simulink model "quadrotor_r2022b"  (R2022b)
settings: Solver=ode4  StartTime=0.0  StopTime=60  FixedStep=1e-3  RelTol=1e-3
libraries: slpidlib x10, dspindex x6, sharedtransform x3, simulink x3, shared6dof x1
(part 2 of 2)

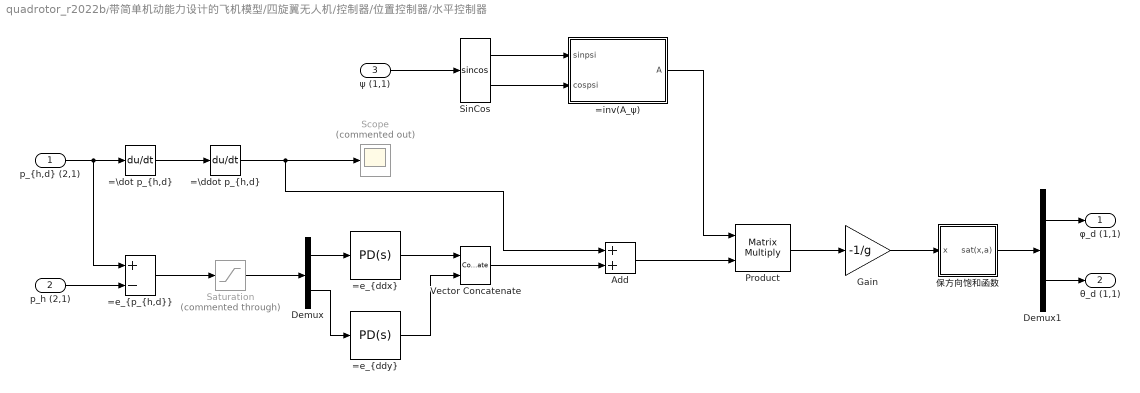
== system quadrotor_r2022b/带简单机动能力设计的飞机模型/四旋翼无人机/控制器/位置控制器/水平控制器 ==
  "p_{h,d} (2,1)" : Inport
  p_h (2,1) : Inport  Port=2
  ψ (1,1) : Inport  Port=3
  "=\\ddot p_{h,d}" : Derivative
  "=\\dot p_{h,d}" : Derivative
  "=e_{ddx}" : slpidlib/PID Controller  Controller=PD  Form=Parallel  TimeDomain=Continuous-time  UseExternalTs=off  SampleTime=-1  IntegratorMethod=Forward Euler  FilterMethod=Forward Euler  ControllerParametersSource=internal  P=K_P_h  I=0  UseKiTs=off  D=K_D_h  N=K_N_h  UseFilter=on  TunerSelectOption=Transfer Function Based (PID Tuner App)  InitialConditionSource=internal  InitialConditionForIntegrator=0  InitialConditionForFilter=0  DifferentiatorICPrevScaledInput=0  ExternalReset=none  TrackingMode=off  Kt=1  LimitOutput=off  SatLimitsSource=internal  UpperSaturationLimit=inf  LowerSaturationLimit=-inf  LinearizeAsGain=on  AntiWindupMode=none  Kb=1  LimitIntegrator=off  UpperIntegratorSaturationLimit=inf  LowerIntegratorSaturationLimit=-inf  POutMin=[]  POutMax=[]  IOutMin=[]  IOutMax=[]  DOutMin=[]  DOutMax=[]  NOutMin=[]  NOutMax=[]  SumOutMin=[]  SumOutMax=[]  SaturationOutMin=[]  SaturationOutMax=[]  PParamMin=[]  PParamMax=[]  IParamMin=[]  IParamMax=[]  DParamMin=[]  DParamMax=[]  NParamMin=[]  NParamMax=[]  KbParamMin=[]  KbParamMax=[]  KtParamMin=[]  KtParamMax=[]  KbOutMin=[]  KbOutMax=[]  KtOutMin=[]  KtOutMax=[]  IntegratorOutMin=[]  IntegratorOutMax=[]  FilterOutMin=[]  FilterOutMax=[]  SumI1OutMin=[]  SumI1OutMax=[]  SumI2OutMin=[]  SumI2OutMax=[]  SumI3OutMin=[]  SumI3OutMax=[]  SumI4OutMin=[]  SumI4OutMax=[]  SumDOutMin=[]  SumDOutMax=[]  DifferentiatorOutMin=[]  DifferentiatorOutMax=[]  FilterDiffOutCoefMin=[]  FilterDiffOutCoefMax=[]  ReciprocalOutMin=[]  ReciprocalOutMax=[]  SumDenOutMin=[]  SumDenOutMax=[]  SumNumOutMin=[]  SumNumOutMax=[]  DivideOutMin=[]  DivideOutMax=[]  UdiffTsProdOutMin=[]  UdiffTsProdOutMax=[]  NTsProdOutMin=[]  NTsProdOutMax=[]  UintegralTsProdOutMin=[]  UintegralTsProdOutMax=[]  UngainTsProdOutMin=[]  UngainTsProdOutMax=[]  ClampingZeroOutDataTypeStr=Inherit: Inherit via back propagation  ClampingZeroOutMin=[]  ClampingZeroOutMax=[]  FilterDenConstantOutDataTypeStr=Inherit: Inherit via back propagation  FilterDenConstantOutMin=[]  FilterDenConstantOutMax=[]  PCopyOutDataTypeStr=Inherit: Inherit via back propagation  PCopyOutMin=[]  PCopyOutMax=[]  NCopyOutDataTypeStr=Inherit: Inherit via back propagation  NCopyOutMin=[]  NCopyOutMax=[]  IntegratorContinuousStateAttributes=''  IntegratorStateMustResolveToSignalObject=off  IntegratorRTWStateStorageClass=Auto  FilterContinuousStateAttributes=''  FilterStateMustResolveToSignalObject=off  FilterRTWStateStorageClass=Auto  ParallelPVariant=InternalParameters  IdealPVariant=Disabled  IVariant=Disabled  DVariant=InternalParameters  IntegratorVariant=Disabled  SatVariant=Disabled  AWVariant=Disabled  PCopyVariant=Disabled  TRVariant=Disabled  FdbkBlocksVariant=Forward  IdealPFdbkVariant=Disabled  SatFdbkVariant=Disabled  DerivativeFilterVariant=ContFilter  NVariant=InternalParameters  NCopyVariant=Disabled  FilterICVariant=InternalICsFilter  IntegratorICVariant=Disabled  ExternalResetVariant=Disabled  TRSumVariant=Passthrough  SumFdbkVariant=Disabled  SumVariant=Sum_PD  TsampFilterVariant=InternalTs  TsampNgainVariant=Passthrough  TsampIntegralVariant=Disabled_SignalSpec  ExternalSaturationOutDataTypeStr=Inherit: Same as second input
  "=e_{ddy}" : slpidlib/PID Controller  Controller=PD  Form=Parallel  TimeDomain=Continuous-time  UseExternalTs=off  SampleTime=-1  IntegratorMethod=Forward Euler  FilterMethod=Forward Euler  ControllerParametersSource=internal  P=K_P_h  I=0  UseKiTs=off  D=K_D_h  N=K_N_h  UseFilter=on  TunerSelectOption=Transfer Function Based (PID Tuner App)  InitialConditionSource=internal  InitialConditionForIntegrator=0  InitialConditionForFilter=0  DifferentiatorICPrevScaledInput=0  ExternalReset=none  TrackingMode=off  Kt=1  LimitOutput=off  SatLimitsSource=internal  UpperSaturationLimit=inf  LowerSaturationLimit=-inf  LinearizeAsGain=on  AntiWindupMode=none  Kb=1  LimitIntegrator=off  UpperIntegratorSaturationLimit=inf  LowerIntegratorSaturationLimit=-inf  POutMin=[]  POutMax=[]  IOutMin=[]  IOutMax=[]  DOutMin=[]  DOutMax=[]  NOutMin=[]  NOutMax=[]  SumOutMin=[]  SumOutMax=[]  SaturationOutMin=[]  SaturationOutMax=[]  PParamMin=[]  PParamMax=[]  IParamMin=[]  IParamMax=[]  DParamMin=[]  DParamMax=[]  NParamMin=[]  NParamMax=[]  KbParamMin=[]  KbParamMax=[]  KtParamMin=[]  KtParamMax=[]  KbOutMin=[]  KbOutMax=[]  KtOutMin=[]  KtOutMax=[]  IntegratorOutMin=[]  IntegratorOutMax=[]  FilterOutMin=[]  FilterOutMax=[]  SumI1OutMin=[]  SumI1OutMax=[]  SumI2OutMin=[]  SumI2OutMax=[]  SumI3OutMin=[]  SumI3OutMax=[]  SumI4OutMin=[]  SumI4OutMax=[]  SumDOutMin=[]  SumDOutMax=[]  DifferentiatorOutMin=[]  DifferentiatorOutMax=[]  FilterDiffOutCoefMin=[]  FilterDiffOutCoefMax=[]  ReciprocalOutMin=[]  ReciprocalOutMax=[]  SumDenOutMin=[]  SumDenOutMax=[]  SumNumOutMin=[]  SumNumOutMax=[]  DivideOutMin=[]  DivideOutMax=[]  UdiffTsProdOutMin=[]  UdiffTsProdOutMax=[]  NTsProdOutMin=[]  NTsProdOutMax=[]  UintegralTsProdOutMin=[]  UintegralTsProdOutMax=[]  UngainTsProdOutMin=[]  UngainTsProdOutMax=[]  ClampingZeroOutDataTypeStr=Inherit: Inherit via back propagation  ClampingZeroOutMin=[]  ClampingZeroOutMax=[]  FilterDenConstantOutDataTypeStr=Inherit: Inherit via back propagation  FilterDenConstantOutMin=[]  FilterDenConstantOutMax=[]  PCopyOutDataTypeStr=Inherit: Inherit via back propagation  PCopyOutMin=[]  PCopyOutMax=[]  NCopyOutDataTypeStr=Inherit: Inherit via back propagation  NCopyOutMin=[]  NCopyOutMax=[]  IntegratorContinuousStateAttributes=''  IntegratorStateMustResolveToSignalObject=off  IntegratorRTWStateStorageClass=Auto  FilterContinuousStateAttributes=''  FilterStateMustResolveToSignalObject=off  FilterRTWStateStorageClass=Auto  ParallelPVariant=InternalParameters  IdealPVariant=Disabled  IVariant=Disabled  DVariant=InternalParameters  IntegratorVariant=Disabled  SatVariant=Disabled  AWVariant=Disabled  PCopyVariant=Disabled  TRVariant=Disabled  FdbkBlocksVariant=Forward  IdealPFdbkVariant=Disabled  SatFdbkVariant=Disabled  DerivativeFilterVariant=ContFilter  NVariant=InternalParameters  NCopyVariant=Disabled  FilterICVariant=InternalICsFilter  IntegratorICVariant=Disabled  ExternalResetVariant=Disabled  TRSumVariant=Passthrough  SumFdbkVariant=Disabled  SumVariant=Sum_PD  TsampFilterVariant=InternalTs  TsampNgainVariant=Passthrough  TsampIntegralVariant=Disabled_SignalSpec  ExternalSaturationOutDataTypeStr=Inherit: Same as second input
  "=e_{p_{h,d}}" : Sum  Inputs=+-
  =inv(A_ψ) : MATLAB Function  TreatAsAtomicUnit=on
  Add : Sum
      settings: AttributesFormatString=|
      | =\ddot{p}+\ddot{e}_{z,d}+K_D*\dot{e}_d+K_P*e_d
      | → \ddot{p} (t→∞)
  Demux : Demux  Outputs=2
  Demux1 : Demux  Outputs=2
  Gain : Gain  Gain=-1/g
  Product : Product  Multiplication=Matrix(*)
  Saturation : Saturate  Commented=through  UpperLimit=1  LowerLimit=-1
      settings: AttributesFormatString=误差限幅，关键
  Scope : Scope  Commented=on
  SinCos : Trigonometry  Operator=sincos
  Vector Concatenate : Concatenate  Mode=Multidimensional array
  保方向饱和函数 : Subsystem  mask{a=pi}
      mask prompts: a "范数上界 (1,1)"
      mask init:
      | assert(a>0,sprintf("expect a>0,but get %f",a))
      mask DialogControl ParameterGroupVar Prompt: 参数
  φ_d (1,1) : Outport
  θ_d (1,1) : Outport  Port=2
  wires:
  "p_{h,d} (2,1)"/1 -> "=e_{p_{h,d}}"/1, "=\\dot p_{h,d}"/1
  "=\\dot p_{h,d}"/1 -> "=\\ddot p_{h,d}"/1
  "=\\ddot p_{h,d}"/1 -> Add/1, Scope/1
  Saturation/1 -> Demux/1
  p_h (2,1)/1 -> "=e_{p_{h,d}}"/2
  "=e_{p_{h,d}}"/1 -> Saturation/1
  ψ (1,1)/1 -> SinCos/1
  Demux/2 -> "=e_{ddy}"/1
  Add/1 -> Product/2
  SinCos/1 -> =inv(A_ψ)/1(sinpsi)
  SinCos/2 -> =inv(A_ψ)/2(cospsi)
  "=e_{ddy}"/1 -> Vector Concatenate/2
  =inv(A_ψ)/1(A) -> Product/1
  Vector Concatenate/1 -> Add/2
  Product/1 -> Gain/1
  Gain/1 -> 保方向饱和函数/1(x)
  保方向饱和函数/1(sat(x,a)) -> Demux1/1
  Demux1/1 -> φ_d (1,1)/1
  Demux1/2 -> θ_d (1,1)/1
  "=e_{ddx}"/1 -> Vector Concatenate/1
  Demux/1 -> "=e_{ddx}"/1

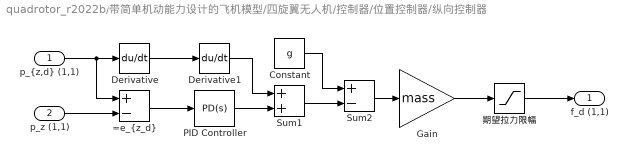
== system quadrotor_r2022b/带简单机动能力设计的飞机模型/四旋翼无人机/控制器/位置控制器/纵向控制器 ==
  "p_{z,d} (1,1)" : Inport
  p_z (1,1) : Inport  Port=2
  "=e_{z_d}" : Sum  Inputs=+-
  Constant : Constant  Value=g  VectorParams1D=off
  Derivative : Derivative
  Derivative1 : Derivative
  Gain : Gain  Gain=mass
  PID Controller : slpidlib/PID Controller  Controller=PD  Form=Parallel  TimeDomain=Continuous-time  UseExternalTs=off  SampleTime=-1  IntegratorMethod=Forward Euler  FilterMethod=Forward Euler  ControllerParametersSource=internal  P=K_P_z  I=0  UseKiTs=off  D=K_D_z  N=K_N_z  UseFilter=on  TunerSelectOption=Transfer Function Based (PID Tuner App)  InitialConditionSource=internal  InitialConditionForIntegrator=0  InitialConditionForFilter=0  DifferentiatorICPrevScaledInput=0  ExternalReset=none  TrackingMode=off  Kt=1  LimitOutput=off  SatLimitsSource=internal  UpperSaturationLimit=inf  LowerSaturationLimit=-inf  LinearizeAsGain=on  AntiWindupMode=none  Kb=1  LimitIntegrator=off  UpperIntegratorSaturationLimit=inf  LowerIntegratorSaturationLimit=-inf  POutMin=[]  POutMax=[]  IOutMin=[]  IOutMax=[]  DOutMin=[]  DOutMax=[]  NOutMin=[]  NOutMax=[]  SumOutMin=[]  SumOutMax=[]  SaturationOutMin=[]  SaturationOutMax=[]  PParamMin=[]  PParamMax=[]  IParamMin=[]  IParamMax=[]  DParamMin=[]  DParamMax=[]  NParamMin=[]  NParamMax=[]  KbParamMin=[]  KbParamMax=[]  KtParamMin=[]  KtParamMax=[]  KbOutMin=[]  KbOutMax=[]  KtOutMin=[]  KtOutMax=[]  IntegratorOutMin=[]  IntegratorOutMax=[]  FilterOutMin=[]  FilterOutMax=[]  SumI1OutMin=[]  SumI1OutMax=[]  SumI2OutMin=[]  SumI2OutMax=[]  SumI3OutMin=[]  SumI3OutMax=[]  SumI4OutMin=[]  SumI4OutMax=[]  SumDOutMin=[]  SumDOutMax=[]  DifferentiatorOutMin=[]  DifferentiatorOutMax=[]  FilterDiffOutCoefMin=[]  FilterDiffOutCoefMax=[]  ReciprocalOutMin=[]  ReciprocalOutMax=[]  SumDenOutMin=[]  SumDenOutMax=[]  SumNumOutMin=[]  SumNumOutMax=[]  DivideOutMin=[]  DivideOutMax=[]  UdiffTsProdOutMin=[]  UdiffTsProdOutMax=[]  NTsProdOutMin=[]  NTsProdOutMax=[]  UintegralTsProdOutMin=[]  UintegralTsProdOutMax=[]  UngainTsProdOutMin=[]  UngainTsProdOutMax=[]  ClampingZeroOutDataTypeStr=Inherit: Inherit via back propagation  ClampingZeroOutMin=[]  ClampingZeroOutMax=[]  FilterDenConstantOutDataTypeStr=Inherit: Inherit via back propagation  FilterDenConstantOutMin=[]  FilterDenConstantOutMax=[]  PCopyOutDataTypeStr=Inherit: Inherit via back propagation  PCopyOutMin=[]  PCopyOutMax=[]  NCopyOutDataTypeStr=Inherit: Inherit via back propagation  NCopyOutMin=[]  NCopyOutMax=[]  IntegratorContinuousStateAttributes=''  IntegratorStateMustResolveToSignalObject=off  IntegratorRTWStateStorageClass=Auto  FilterContinuousStateAttributes=''  FilterStateMustResolveToSignalObject=off  FilterRTWStateStorageClass=Auto  ParallelPVariant=InternalParameters  IdealPVariant=Disabled  IVariant=Disabled  DVariant=InternalParameters  IntegratorVariant=Disabled  SatVariant=Disabled  AWVariant=Disabled  PCopyVariant=Disabled  TRVariant=Disabled  FdbkBlocksVariant=Forward  IdealPFdbkVariant=Disabled  SatFdbkVariant=Disabled  DerivativeFilterVariant=ContFilter  NVariant=InternalParameters  NCopyVariant=Disabled  FilterICVariant=InternalICsFilter  IntegratorICVariant=Disabled  ExternalResetVariant=Disabled  TRSumVariant=Passthrough  SumFdbkVariant=Disabled  SumVariant=Sum_PD  TsampFilterVariant=InternalTs  TsampNgainVariant=Passthrough  TsampIntegralVariant=Disabled_SignalSpec  ExternalSaturationOutDataTypeStr=Inherit: Same as second input
  Sum1 : Sum
      settings: AttributesFormatString=|
      | =\ddot{p}+\ddot{e}_{z,d}+K_D*\dot{e}_d+K_P*e_d
      | → \ddot{p} (t→∞)
  Sum2 : Sum  Inputs=+-
  期望拉力限幅 : Saturate  UpperLimit=f_max  LowerLimit=f_min
  f_d (1,1) : Outport
  wires:
  "p_{z,d} (1,1)"/1 -> Derivative/1, "=e_{z_d}"/1
  期望拉力限幅/1 -> f_d (1,1)/1
  Gain/1 -> 期望拉力限幅/1
  p_z (1,1)/1 -> "=e_{z_d}"/2
  Constant/1 -> Sum2/1
  Derivative/1 -> Derivative1/1
  Sum2/1 -> Gain/1
  Derivative1/1 -> Sum1/1
  Sum1/1 -> Sum2/2
  PID Controller/1 -> Sum1/2
  "=e_{z_d}"/1 -> PID Controller/1

== system quadrotor_r2022b/带简单机动能力设计的飞机模型/四旋翼无人机/控制器/姿态控制器/mod ==
  x : Inport
  Add : Sum  Inputs=+-
  Add1 : Sum  Inputs=+-
  Constant : Constant  Value=a  VectorParams1D=off
  Floor : Rounding
  Product : Product  Inputs=*/
  Product1 : Product
  m : Constant  Value=b-a  VectorParams1D=off
  x mod [a,b) : Outport
  wires:
  x/1 -> Add/1, Add1/1
  Product/1 -> Floor/1
  Add/1 -> Product/1
  Constant/1 -> Add/2
  m/1 -> Product1/2, Product/2
  Product1/1 -> Add1/2
  Floor/1 -> Product1/1
  Add1/1 -> x mod [a,b)/1

== system quadrotor_r2022b/带简单机动能力设计的飞机模型/四旋翼无人机/控制器/姿态控制器（旋转矩阵版）/mod ==
  x : Inport
  Add : Sum  Inputs=+-
  Add1 : Sum  Inputs=+-
  Constant : Constant  Value=a  VectorParams1D=off
  Floor : Rounding
  Product : Product  Inputs=*/
  Product1 : Product
  m : Constant  Value=b-a  VectorParams1D=off
  x mod [a,b) : Outport
  wires:
  x/1 -> Add/1, Add1/1
  Product/1 -> Floor/1
  Add/1 -> Product/1
  Constant/1 -> Add/2
  m/1 -> Product1/2, Product/2
  Product1/1 -> Add1/2
  Floor/1 -> Product1/1
  Add1/1 -> x mod [a,b)/1

== system quadrotor_r2022b/带简单机动能力设计的飞机模型/四旋翼无人机/控制器/位置控制器/水平控制器/保方向饱和函数 ==
  x : Inport
  Abs : Abs  SaturateOnIntegerOverflow=off
  Constant : Constant  Value=a
  Constant1 : Constant
  Divide : Product  Inputs=*/
  Max : MinMax  Inputs=2
  MinMax : MinMax  Function=max
  Product : Product
  Switch : Switch  Criteria=u2 > Threshold  SaturateOnIntegerOverflow=off  InputSameDT=off
  sat(x,a) : Outport
  wires:
  x/1 -> Product/1, Abs/1
  Abs/1 -> MinMax/1
  MinMax/1 -> Switch/2, Switch/1
  Constant/1 -> Divide/1, Switch/3
  Switch/1 -> Divide/2
  Constant1/1 -> Max/2
  Divide/1 -> Max/1
  Max/1 -> Product/2
  Product/1 -> sat(x,a)/1

== matlab function quadrotor_r2022b/带简单机动能力设计的飞机模型/四旋翼无人机/控制器/姿态控制器（旋转矩阵版）/MATLAB Function ==
  data: A input; A_vee output
function A_vee = vex(A)
% x^\wedge 逆运算
A_vee = [A(3,2);A(1,3);A(2,1)];

== matlab function quadrotor_r2022b/带简单机动能力设计的飞机模型/四旋翼无人机/控制器/位置控制器/水平控制器/=inv(A_ψ) ==
  data: sinpsi input; cospsi input; A output
function A = fcn(sinpsi,cospsi)
A=[
    sinpsi,-cospsi;
    cospsi,sinpsi];
end
